simulink model "sis_dinamico1"  (R2021a)
settings: Solver=VariableStepAuto  StartTime=0.0  StopTime=50  RelTol=1e-3
settings Model: Creator=GIOVANNI  LastModifiedBy=GIOVANNI
settings SolverCC: AlgebraicLoopSolver=TrustRegion
settings DebuggingCC: SFMachineParentedDataDiag=warning

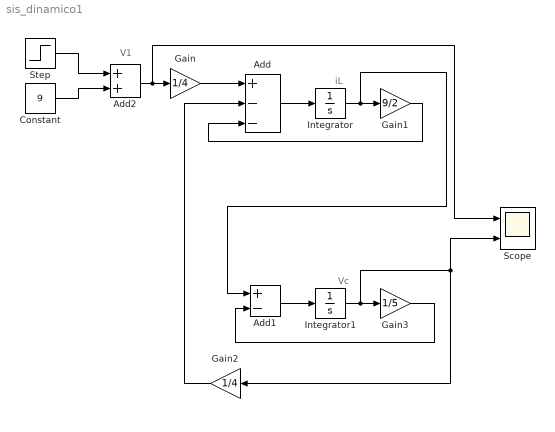
== system sis_dinamico1 ==
  note: Vc
  note: iL
  note: V1
  Add : Sum  Inputs=+--
  Add1 : Sum  Inputs=+-
  Add2 : Sum
  Constant : Constant  Value=9
  Gain : Gain  Gain=1/4
  Gain1 : Gain  Gain=9/2
  Gain2 : Gain  Gain=1/4
  Gain3 : Gain  Gain=1/5
  Integrator : Integrator
  Integrator1 : Integrator
  Scope : Scope  NumInputPorts=2
  Step : Step  Time=5  SampleTime=0
  wires:
  Step/1 -> Add2/1
  Constant/1 -> Add2/2
  Add2/1 -> Scope/1, Gain/1
  Gain/1 -> Add/1
  Add/1 -> Integrator/1
  Integrator/1 -> Gain1/1, Add1/1
  Gain2/1 -> Add/2
  Add1/1 -> Integrator1/1
  Integrator1/1 -> Gain3/1, Gain2/1, Scope/2
  Gain3/1 -> Add1/2
  Gain1/1 -> Add/3
